simulink model "pva2"  (R2019b)
settings: Solver=FixedStepAuto  StartTime=0.0  StopTime=30  FixedStep=0.01  RelTol=1e-3
settings Model: Creator=suvo  LastModifiedBy=suvo

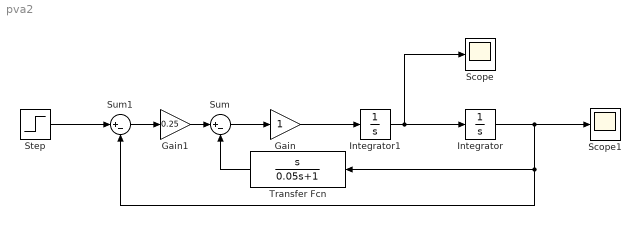
== system pva2 ==
  Gain : Gain
  Gain1 : Gain  Gain=0.25
  Integrator : Integrator
  Integrator1 : Integrator
  Scope : Scope
  Scope1 : Scope
  Step : Step  SampleTime=0
  Sum : Sum  Inputs=|+-
  Sum1 : Sum  Inputs=|+-
  Transfer Fcn : TransferFcn  Numerator=[1 0]  Denominator=[0.05 1]
  wires:
  Sum/1 -> Gain/1
  Gain/1 -> Integrator1/1
  Integrator1/1 -> Integrator/1, Scope/1
  Sum1/1 -> Gain1/1
  Integrator/1 -> Scope1/1, Transfer Fcn/1, Sum1/2
  Transfer Fcn/1 -> Sum/2
  Step/1 -> Sum1/1
  Gain1/1 -> Sum/1
